simulink model "rasberrypi_publish_subscribe"  (R2020a)
settings: Solver=FixedStepAuto  StartTime=0.0  StopTime=inf  RelTol=1e-3  EnableMultiTasking=on
PreLoadFcn:
  | Ts = 0.01;
model workspace (MAT data in the model file):
  SL_ROS_VariableLengthArrays_MaxSizes.CommonInfo.ArrayTruncateAction = 'EmitWarning'
  SL_ROS_VariableLengthArrays_MaxSizes.MsgTypeMap = containers.Map
  SL_ROS_VariableLengthArrays_MaxSizes.MsgTypeMap.serialization.keys = {'sensor_msgs/Image'}
  SL_ROS_VariableLengthArrays_MaxSizes.MsgTypeMap.serialization.values{1}(1).PropertyName = 'Data'
  SL_ROS_VariableLengthArrays_MaxSizes.MsgTypeMap.serialization.values{1}(1).DataType = 'uint8'
  SL_ROS_VariableLengthArrays_MaxSizes.MsgTypeMap.serialization.values{1}(1).MaxLength = 57600
  SL_ROS_VariableLengthArrays_MaxSizes.MsgTypeMap.serialization.values{1}(2).PropertyName = 'Encoding'
  SL_ROS_VariableLengthArrays_MaxSizes.MsgTypeMap.serialization.values{1}(2).DataType = 'uint8'
  SL_ROS_VariableLengthArrays_MaxSizes.MsgTypeMap.serialization.values{1}(2).MaxLength = 4
  SL_ROS_VariableLengthArrays_MaxSizes.MsgTypeMap.serialization.uniformity = 0
  SL_ROS_VariableLengthArrays_MaxSizes.MsgTypeMap.serialization.keyType = 'char'
  SL_ROS_VariableLengthArrays_MaxSizes.MsgTypeMap.serialization.valueType = 'any'
libraries: robotlib x6, simulink x2, visiontextngfix x1, raspberrypilib x1, embdlinuxlib x1
settings Model: Creator=The MathWorks, Inc.  LastModifiedBy=mmordeka
settings SolverCC: AutoInsertRateTranBlk=on
settings DataIOCC: SaveFormat=Array  ReturnWorkspaceOutputs=off
settings OptimizationCC: ZeroExternalMemoryAtStartup=off  ZeroInternalMemoryAtStartup=off  LifeSpan=Inf  MaxStackSize=64  EfficientTunableParamExpr=on
settings DebuggingCC: SolverPrmCheckMsg=warning  AllowSymbolicDim=off  SFUnexpectedBacktrackingDiag=warning  SFNoUnconditionalDefaultTransitionDiag=warning  SFExecutionAtInitializationDiag=none  ArithmeticOperatorsInVariantConditions=warning
settings HardwareCC: ProdBitPerPointer=32  ProdBitPerSizeT=32  ProdBitPerPtrDiffT=32  ProdLargestAtomicInteger=Long  ProdLargestAtomicFloat=Double  ProdWordSize=32  ProdHWDeviceType=ARM Compatible->ARM Cortex
settings ModelReferenceCC: PropagateSignalLabelsOutOfModel=off
settings SFSimCC: SimUseLocalCustomCode=off  MATLABDynamicMemAlloc=off  CustomCodeUndefinedFunction=UseInterfaceOnly
settings RTWCC: SystemTargetFile=ert.tlc  HardwareBoard=Raspberry Pi - Robot Operating System (ROS)  TemplateMakefile=ert_default_tmf  GenerateReport=on  RTWUseLocalCustomCode=off  Toolchain=Catkin  IncludeHyperlinkInReport=on  LaunchReport=on  TargetLang=C++  GenerateTraceInfo=on  GenerateTraceReport=on  GenerateTraceReportSl=on  GenerateTraceReportSf=on  GenerateTraceReportEml=on
settings CodeAppCC: ForceParamTrailComments=on  OperatorAnnotations=on  SimulinkDataObjDesc=on  SFDataObjDesc=on  MATLABFcnDesc=on  InsertBlockDesc=on  StateflowObjectComments=on  MATLABSourceComments=on
settings ERTTargetCC: MultiwordLength=2048  MultiInstanceERTCode=on  CodeInterfacePackaging=C++ class  SupportVariableSizeSignals=on  RootIOFormat=Structure reference
settings ConfigComp: CovMetricSettings=dw  CovHtmlReporting=on  CovSaveCumulativeToWorkspaceVar=on  CovSaveSingleToWorkspaceVar=on  CovExternalEMLEnable=off  CovSFcnEnable=off

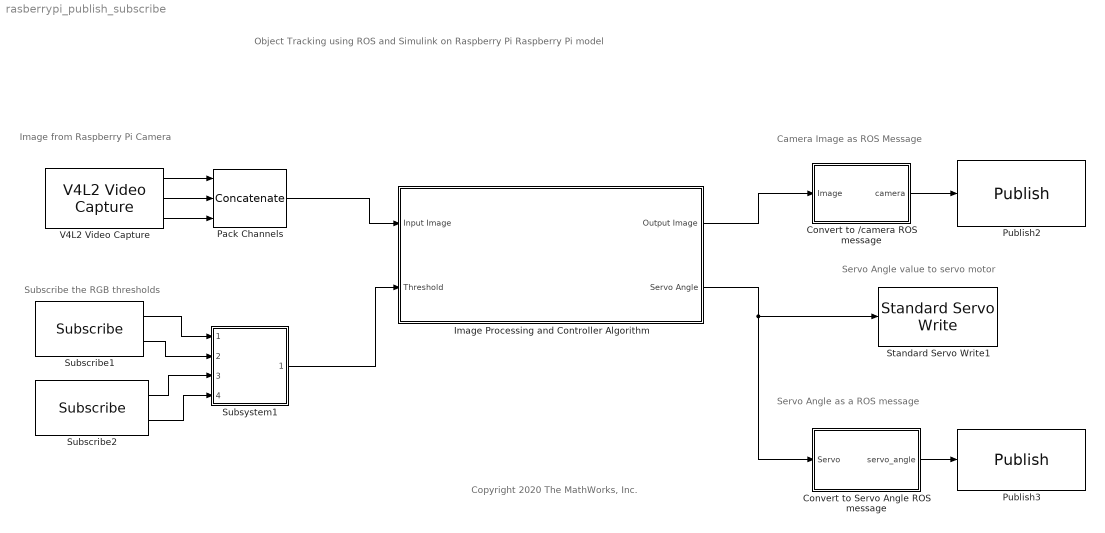
== system rasberrypi_publish_subscribe ==
  note: Servo Angle value to servo motor
  note: Subscribe the RGB thresholds
  note: Image from Raspberry Pi Camera
  note: Camera Image as ROS Message
  note: Servo Angle as a ROS message
  note: Object Tracking using ROS and Simulink on Raspberry Pi
      | Raspberry Pi model
  note: Copyright 2020 The MathWorks, Inc.
  Convert to /camera ROS message : Subsystem
  Convert to Servo Angle ROS message : Subsystem
  Image Processing and Controller Algorithm : Subsystem
  Pack Channels : Concatenate  NumInputs=3  Mode=Multidimensional array  ConcatenateDimension=3
  Publish2 : robotlib/Publish  topicSource=Specify your own  topic=/camera  messageType=sensor_msgs/Image  messageQueueLength=1
  Publish3 : robotlib/Publish  topicSource=Specify your own  topic=/servo_angle  messageType=std_msgs/UInt8  messageQueueLength=1
  Standard Servo Write1 : raspberrypilib/Standard Servo Write  board=Pi 3 Model B  Pin_=18  MinPulseDuration=1000e-6  MaxPulseDuration=2000e-6  blockPlatform=Raspberry Pi
      settings: SourceProductBaseCode=RASPPI
  Subscribe1 : robotlib/Subscribe  topicSource=Specify your own  topic=/minRGBThreshold  messageType=std_msgs/ColorRGBA  sampleTime=Ts  messageQueueLength=51
  Subscribe2 : robotlib/Subscribe  topicSource=Specify your own  topic=/maxRGBThreshold  messageType=std_msgs/ColorRGBA  sampleTime=Ts  messageQueueLength=51
  Subsystem1 : Subsystem
  V4L2 Video Capture : embdlinuxlib/V4L2 Video Capture  m_devName='/dev/video0'  roi=[0, 0, 640, 480]  imSizeSelection=160x120  imSize=[640, 480]  pixelFormat=RGB  pixelOrder=Planar  sampleTime=Ts  simOutput=Colorbars  blockPlatform=Raspberry Pi
      settings: SourceProductBaseCode=SC_BEAGLEBONE_BLUE,RASPPI
  wires:
  V4L2 Video Capture/1 -> Pack Channels/1
  V4L2 Video Capture/2 -> Pack Channels/2
  V4L2 Video Capture/3 -> Pack Channels/3
  Pack Channels/1 -> Image Processing and Controller Algorithm/1(Input Image)
  Subscribe1/1 -> Subsystem1/1(EnableMin)
  Subscribe1/2 -> Subsystem1/2(MinRGB)
  Subscribe2/1 -> Subsystem1/3(EnableMax)
  Subscribe2/2 -> Subsystem1/4(MaxRGB)
  Subsystem1/1(threshold) -> Image Processing and Controller Algorithm/2(Threshold)
  Image Processing and Controller Algorithm/1(Output Image) -> Convert to /camera ROS message/1(Image)
  Image Processing and Controller Algorithm/2(Servo Angle) -> Convert to Servo Angle ROS message/1(Servo), Standard Servo Write1/1
  Convert to Servo Angle ROS message/1(servo_angle) -> Publish3/1
  Convert to /camera ROS message/1(camera) -> Publish2/1

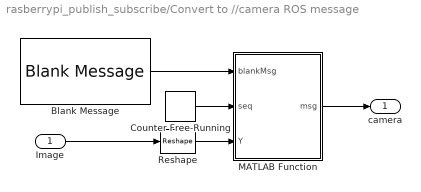
== system rasberrypi_publish_subscribe/Convert to //camera ROS message ==
  Image : Inport
  Blank Message : robotlib/Blank Message  messageClass=Message  entityType=sensor_msgs/Image  messageType=sensor_msgs/Image  SampleTime=Ts
  Counter Free-Running : simulink/Sources/Counter Free-Running  NumBits=32  tsamp=-1
  MATLAB Function : MATLAB Function  TreatAsAtomicUnit=on
  Reshape : Reshape
  camera : Outport
  wires:
  MATLAB Function/1(msg) -> camera/1
  Counter Free-Running/1 -> MATLAB Function/2(seq)
  Reshape/1 -> MATLAB Function/3(Y)
  Blank Message/1 -> MATLAB Function/1(blankMsg)
  Image/1 -> Reshape/1

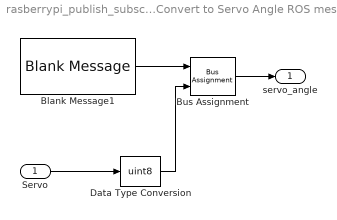
== system rasberrypi_publish_subscribe/Convert to Servo Angle ROS message ==
  Servo : Inport
  Blank Message1 : robotlib/Blank Message  messageClass=Message  entityType=std_msgs/UInt8  messageType=std_msgs/UInt8  SampleTime=inf
  Bus Assignment : BusAssignment  AssignedSignals=Data
  Data Type Conversion : DataTypeConversion  OutDataTypeStr=uint8
  servo_angle : Outport
  wires:
  Blank Message1/1 -> Bus Assignment/1
  Data Type Conversion/1 -> Bus Assignment/2
  Bus Assignment/1 -> servo_angle/1
  Servo/1 -> Data Type Conversion/1

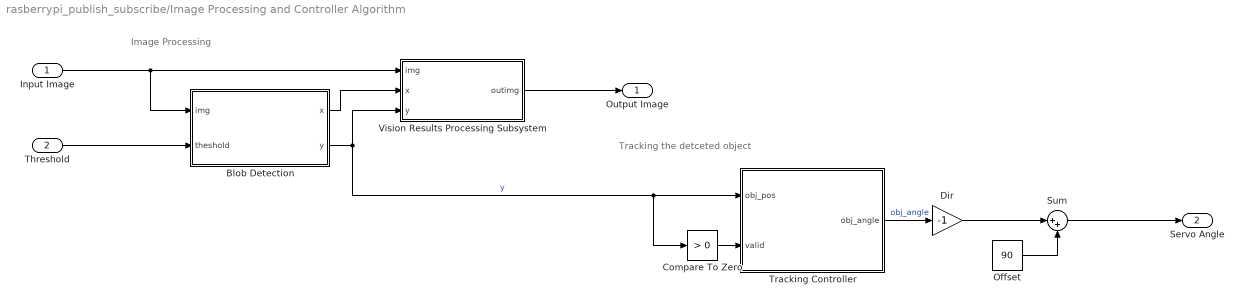
== system rasberrypi_publish_subscribe/Image Processing and Controller Algorithm ==
  note: Tracking the detceted object
  note: Image Processing
  Input Image : Inport
  Threshold : Inport  Port=2
  Blob Detection : Subsystem
  Compare To Zero : simulink/Logic and Bit Operations/Compare To Zero  relop=>  OutDataTypeStr=boolean  ZeroCross=off
  Dir : Gain  Gain=-1
  Offset : Constant  Value=90  SampleTime=Ts
  Sum : Sum  Inputs=|++
  Tracking Controller : Stateflow chart  TreatAsAtomicUnit=on
  Vision Results Processing Subsystem : Subsystem
  Output Image : Outport
  Servo Angle : Outport  Port=2
  wires:
  Offset/1 -> Sum/2
  Sum/1 -> Servo Angle/1
  Blob Detection/1(x) -> Vision Results Processing Subsystem/2(x)
  Compare To Zero/1 -> Tracking Controller/2(valid)
  Input Image/1 -> Blob Detection/1(img), Vision Results Processing Subsystem/1(img)
  Threshold/1 -> Blob Detection/2(theshold)
  Tracking Controller/1(obj_angle) -> Dir/1  "obj_angle"
  Blob Detection/2(y) -> Vision Results Processing Subsystem/3(y), Compare To Zero/1, Tracking Controller/1(obj_pos)  "y"
  Dir/1 -> Sum/1
  Vision Results Processing Subsystem/1(outimg) -> Output Image/1

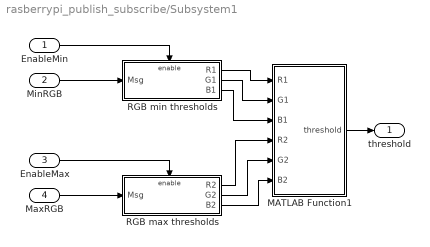
== system rasberrypi_publish_subscribe/Subsystem1 ==
  EnableMin : Inport
  MinRGB : Inport  Port=2
  EnableMax : Inport  Port=3
  MaxRGB : Inport  Port=4
  MATLAB Function1 : MATLAB Function  TreatAsAtomicUnit=on
  RGB max thresholds : Subsystem
  RGB min thresholds : Subsystem
  threshold : Outport
  wires:
  RGB min thresholds/3(B1) -> MATLAB Function1/3(B1)
  RGB max thresholds/2(G2) -> MATLAB Function1/5(G2)
  RGB max thresholds/1(R2) -> MATLAB Function1/4(R2)
  MinRGB/1 -> RGB min thresholds/1(Msg)
  MaxRGB/1 -> RGB max thresholds/1(Msg)
  MATLAB Function1/1(threshold) -> threshold/1
  RGB min thresholds/1(R1) -> MATLAB Function1/1(R1)
  RGB max thresholds/3(B2) -> MATLAB Function1/6(B2)
  RGB min thresholds/2(G1) -> MATLAB Function1/2(G1)
  EnableMin/1 -> RGB min thresholds/Enable
  EnableMax/1 -> RGB max thresholds/Enable

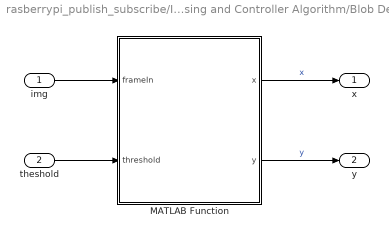
== system rasberrypi_publish_subscribe/Image Processing and Controller Algorithm/Blob Detection ==
  img : Inport  OutDataTypeStr=uint8  PortDimensions=[160 120 3]
  theshold : Inport  Port=2
  MATLAB Function : MATLAB Function  TreatAsAtomicUnit=on
  x : Outport  OutDataTypeStr=double  PortDimensions=1  VectorParamsAs1DForOutWhenUnconnected=off
  y : Outport  Port=2  OutDataTypeStr=double  PortDimensions=1  VectorParamsAs1DForOutWhenUnconnected=off
  wires:
  img/1 -> MATLAB Function/1(frameIn)
  MATLAB Function/1(x) -> x/1  "x"
  MATLAB Function/2(y) -> y/1  "y"
  theshold/1 -> MATLAB Function/2(threshold)

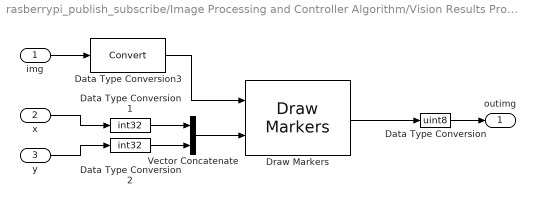
== system rasberrypi_publish_subscribe/Image Processing and Controller Algorithm/Vision Results Processing Subsystem ==
  img : Inport
  x : Inport  Port=2
  y : Inport  Port=3
  Data Type Conversion : DataTypeConversion  OutDataTypeStr=uint8
  Data Type Conversion1 : DataTypeConversion  OutDataTypeStr=int32
  Data Type Conversion2 : DataTypeConversion  OutDataTypeStr=int32
  Data Type Conversion3 : DataTypeConversion
  Draw Markers : visiontextngfix/Draw Markers  shape=Circle  size=3  fill=off  fillClrSource=Specify via dialog  display=Black  intensity=200  color=[200 255 100]  opacity=0.6  viewport=Entire image  antialiasing=off  inType=Obsolete  imagePorts=One multidimensional signal  roundingMode=Floor  overflowMode=off  memoryMode=Specify word length  memoryWordLength=16  memoryFracLength=15  prodOutputMode=Binary point scaling  prodOutputWordLength=32  prodOutputFracLength=14
      settings: SourceProductBaseCode=VP
  Vector Concatenate : Concatenate
  outimg : Outport  VectorParamsAs1DForOutWhenUnconnected=off
  wires:
  Data Type Conversion3/1 -> Draw Markers/1
  Vector Concatenate/1 -> Draw Markers/2
  Data Type Conversion2/1 -> Vector Concatenate/2
  Draw Markers/1 -> Data Type Conversion/1
  Data Type Conversion1/1 -> Vector Concatenate/1
  y/1 -> Data Type Conversion2/1
  img/1 -> Data Type Conversion3/1
  x/1 -> Data Type Conversion1/1
  Data Type Conversion/1 -> outimg/1

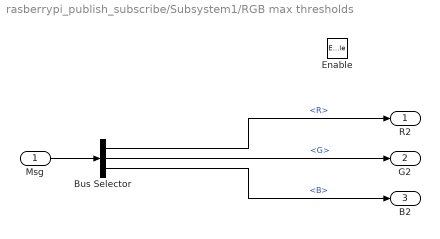
== system rasberrypi_publish_subscribe/Subsystem1/RGB max thresholds ==
  Msg : Inport
  Enable : EnablePort
  Bus Selector : BusSelector  OutputSignals=R,G,B
  R2 : Outport
  G2 : Outport  Port=2
  B2 : Outport  Port=3
  wires:
  Msg/1 -> Bus Selector/1
  Bus Selector/1 -> R2/1  "<R>"
  Bus Selector/3 -> B2/1  "<B>"
  Bus Selector/2 -> G2/1  "<G>"

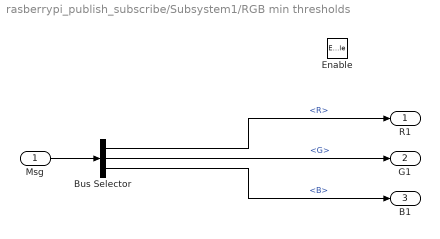
== system rasberrypi_publish_subscribe/Subsystem1/RGB min thresholds ==
  Msg : Inport
  Enable : EnablePort
  Bus Selector : BusSelector  OutputSignals=R,G,B
  R1 : Outport
  G1 : Outport  Port=2
  B1 : Outport  Port=3
  wires:
  Msg/1 -> Bus Selector/1
  Bus Selector/1 -> R1/1  "<R>"
  Bus Selector/3 -> B1/1  "<B>"
  Bus Selector/2 -> G1/1  "<G>"

== matlab function rasberrypi_publish_subscribe/Image Processing and Controller Algorithm/Blob Detection/MATLAB Function ==
  data: x output; frameIn input uint8 size=[160 120 3]; y output; threshold input
function [x,y] = detectROI(frameIn, threshold)
%#Codegen 

% This funtcion thresholds the image based on threshold values submitted by
% the user

%% Setup the detector and initialize variables
persistent detector 
if isempty(detector)
    detector = vision.BlobAnalysis('BoundingBoxOutputPort',false,...
        'AreaOutputPort',false,'MinimumBlobArea',300, ...
        'MajorAxisLengthOutputPort',true,'MaximumCount', 10);
end
x = 0;
y = 0;

%% Threshold the image
%frameIn = rgb2ycbcr(frameIn);
mask = (frameIn (:,:,1) >= threshold(1,1))& (frameIn (:,:,1) <= threshold(1,2))&...
    (frameIn (:,:,2) >= threshold(2,1))& (frameIn (:,:,2) <= threshold(2,2))&...
    (frameIn (:,:,3) >= threshold(3,1))& (frameIn (:,:,3) <= threshold(3,2));

[centroid,majorAxis] = detector(mask);


if ~isempty(majorAxis)
% Identify Largest Blob
    [~,mIdx] = max(majorAxis);
    C = centroid(mIdx,:);
    x = double(C(1));
    y = double(C(2));

end 

end

== stateflow chart rasberrypi_publish_subscribe/Image Processing and Controller Algorithm/Tracking Controller ==
  settings: sampleTime=1/15  executeAtInitialization=1
  state dir = setDir(position) [function]
    (default) -> (junction 102)
    (junction 102) -> (junction 119) [order 1] : [position > 160]
    (junction 102) -> (junction 107) [order 2] : {dir = -1}
    (junction 119) -> (junction 105) : {dir = 1}
    (junction 105) -> (junction 107)
    (junction 107) -> (junction 96)
  state Tracking
    entry,during:
    obj_angle = objAngle(obj_pos)*50;
    direction = setDir(obj_pos);
  state Waiting
    entry:
    i =0;
    during:
    i = i + 1;
  state Seeking
    Seeking -> (junction 120) [order 1]
    (junction 120) -> (junction 98) [order 2]
    (junction 120) -> (junction 97) [order 1] : [direction==1]
    (junction 97) -> (junction 121) [order 2] : {direction=-1;}
    (junction 98) -> (junction 108) [order 2] : {direction=1;}
    (junction 97) -> (junction 121) [order 1] : [obj_angle < MAX_ANGLE]
        | {obj_angle = obj_angle + 5;}
    (junction 98) -> (junction 108) [order 1] : [obj_angle>-MAX_ANGLE]
        | {obj_angle = obj_angle - 5;}
    (junction 108) -> (junction 122)
    (junction 121) -> (junction 122)
  (default) -> Tracking
  Tracking -> Waiting : [~valid]
  Waiting -> Tracking [order 2] : [valid]
  Waiting -> Seeking [order 1] : [i>5]
  Seeking -> Tracking [order 1] : [valid]
  data: position function_input double; dir function_output double; pos function_input double; a function_output double; obj_pos input double; MAX_ANGLE local double =90; valid input; i local double; obj_angle output double; direction local double
  function a = objAngle(pos):
    | function a = objAngle(pos)
    | 
    | % a = atand((pos-200)/5000);
    | deadZone = 0.2;
    | 
    | a =(pos - 160)/160;
    | 
    | if abs(a)<(deadZone/2)
    |    a=0;
    | end
    | 
    | 
    | end

== matlab function rasberrypi_publish_subscribe/Subsystem1/MATLAB Function1 ==
  data: R1 input; threshold output; G1 input; B1 input; R2 input; G2 input; B2 input
function threshold = fcn(R1, G1, B1, R2, G2, B2)

threshold = [R1 R2; G1 G2; B1 B2];

== matlab function rasberrypi_publish_subscribe/Convert to //camera ROS message/MATLAB Function ==
  data: blankMsg input Bus: SL_Bus_rasberrypi_publish_subscribe_sensor_msgs_Image; seq input; msg output Bus: SL_Bus_rasberrypi_publish_subscribe_sensor_msgs_Image; Y input
function msg = fcn(blankMsg, seq,Y)
%#codegen

% Set width and height 
msg = blankMsg;
msg.Width = uint32(160);
msg.Height = uint32(120);

% Black and white image
msg.Encoding_SL_Info.CurrentLength = uint32(4);
msg.Encoding = uint8('rgb8')';

% Size of image buffer = 160 * 120
msg.Data_SL_Info.CurrentLength = uint32(57600);
msg.Data = Y;

% Sequence number
msg.Header.Seq = seq;
end
